simulink model "Cruise_control"  (R2020b)
settings: Solver=VariableStepAuto  StartTime=0.0  StopTime=10.0  RelTol=1e-3
undefined symbols (not defined in the file or in its folder): b, Kd, Ki, Kp, m
settings Model: DataDictionary=Cruise_control_data.sldd  Creator=JAGRUTI SHINDE  LastModifiedBy=JAGRUTI SHINDE

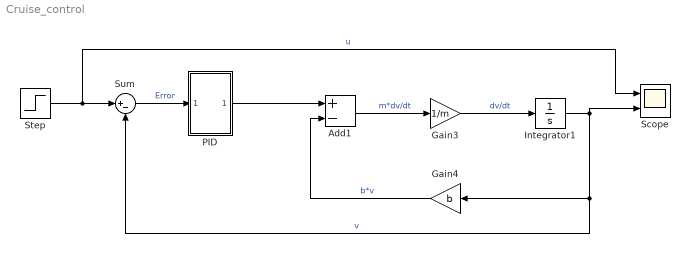
== system Cruise_control ==
  Add1 : Sum  Inputs=+-
  Gain3 : Gain  Gain=1/m
  Gain4 : Gain  Gain=b
  Integrator1 : Integrator
  "PID " : Subsystem
  Scope : Scope  NumInputPorts=2
  Step : Step  SampleTime=0
  Sum : Sum  Inputs=|+-
  wires:
  Step/1 -> Scope/1, Sum/1  "u"
  Add1/1 -> Gain3/1  "m*dv/dt"
  Gain3/1 -> Integrator1/1  "dv/dt"
  Integrator1/1 -> Gain4/1, Sum/2, Scope/2  "v"
  Gain4/1 -> Add1/2  "b*v"
  Sum/1 -> "PID "/1(In1)  "Error"
  "PID "/1(Out1) -> Add1/1

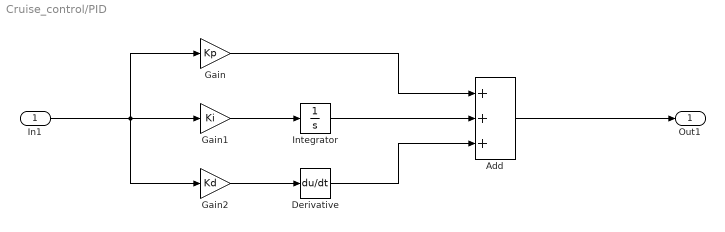
== system Cruise_control/PID  ==
  In1 : Inport
  Add : Sum  Inputs=+++
  Derivative : Derivative
  Gain : Gain  Gain=Kp
  Gain1 : Gain  Gain=Ki
  Gain2 : Gain  Gain=Kd
  Integrator : Integrator
  Out1 : Outport
  wires:
  Add/1 -> Out1/1
  Gain/1 -> Add/1
  Gain2/1 -> Derivative/1
  Integrator/1 -> Add/2
  Gain1/1 -> Integrator/1
  Derivative/1 -> Add/3
  In1/1 -> Gain/1, Gain2/1, Gain1/1
